simulink model "bh_2dof_STARTING_POINT_MODEL_SIMULINK"  (R2017a)
settings: Solver=ode45  StartTime=0.0  StopTime=20  RelTol=1e-5  EnableMultiTasking=on
settings Model: Creator=bhorton  LastModifiedBy=bhorton
settings OptimizationCC: LifeSpan=inf
settings DebuggingCC: SFUnexpectedBacktrackingDiag=warning  SFNoUnconditionalDefaultTransitionDiag=warning  SFExecutionAtInitializationDiag=none
settings GRTTargetCC: TargetLangStandard=C89/C90 (ANSI)  GeneratePreprocessorConditionals=Disable all
settings ConfigComp: CovMetricSettings=dw  CovHtmlReporting=on  CovSaveCumulativeToWorkspaceVar=on  CovSaveSingleToWorkspaceVar=on  CovExternalEMLEnable=off

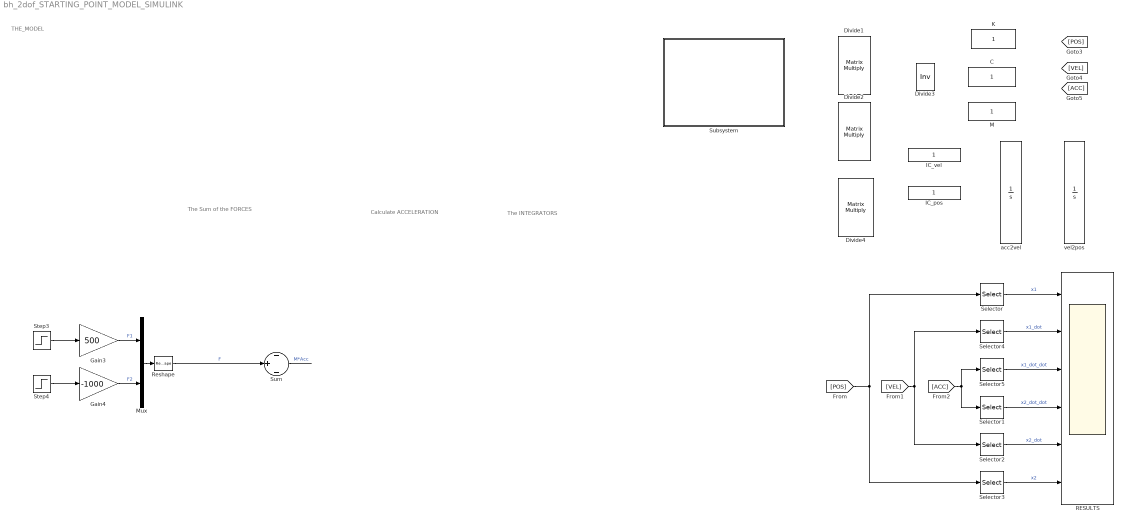
== system bh_2dof_STARTING_POINT_MODEL_SIMULINK ==
  note: The Sum of the FORCES
  note: Calculate ACCELERATION
  note: The INTEGRATORS
  note: THE_MODEL
  C : Constant
  Divide1 : Product  Multiplication=Matrix(*)
  Divide2 : Product  Multiplication=Matrix(*)
  Divide3 : Product  Inputs=/  Multiplication=Matrix(*)
  Divide4 : Product  Multiplication=Matrix(*)
  Gain3 : Gain  Gain=500
  Gain4 : Gain  Gain=-1000
  IC_pos : Constant
  IC_vel : Constant
  K : Constant
  M : Constant
  Mux : Mux  Inputs=2
  RESULTS : Scope  NumInputPorts=6
  Reshape : Reshape  OutputDimensionality=Column vector (2-D)
  Selector : Selector  InputPortWidth=2  IndexOptions=Index vector (dialog)  Indices=[1 ]  OutputSizes=1
  Selector1 : Selector  InputPortWidth=2  IndexOptions=Index vector (dialog)  Indices=[2]  OutputSizes=1
  Selector2 : Selector  InputPortWidth=2  IndexOptions=Index vector (dialog)  Indices=[2]  OutputSizes=1
  Selector3 : Selector  InputPortWidth=2  IndexOptions=Index vector (dialog)  Indices=[2]  OutputSizes=1
  Selector4 : Selector  InputPortWidth=2  IndexOptions=Index vector (dialog)  Indices=[1 ]  OutputSizes=1
  Selector5 : Selector  InputPortWidth=2  IndexOptions=Index vector (dialog)  Indices=[1 ]  OutputSizes=1
  Step3 : Step  Time=5  SampleTime=0
      settings: AttributesFormatString=Step @ T=%<Time>
  Step4 : Step  Time=10  SampleTime=0
      settings: AttributesFormatString=Step @ T=%<Time>
  Subsystem : Subsystem
      mask init:
      | str1 = 'Double click me';
      | str2 = 'to load MODEL';
      | str3 = 'parameters into';
      | str4 = 'Workspace';
      settings: OpenFcn=|
      | clc;
      | bh_script_2dof_params;
      | whos
      | fprintf('\n %s', repmat('#',1,70));
      | fprintf('\n DONE ! \n')
      mask Display: fprintf('%s\n%s\n%s\n%s',str1,str2,str3,str4)
  Sum : Sum  Inputs=-|+|-
  acc2vel : Integrator  InitialConditionSource=external
  vel2pos : Integrator  InitialConditionSource=external
  wires:
  Selector4/1 -> RESULTS/2  "x1_dot"
  [ACC] -> Selector5/1, Selector1/1
  Selector5/1 -> RESULTS/3  "x1_dot_dot"
  Selector/1 -> RESULTS/1  "x1"
  Mux/1 -> Reshape/1
  Reshape/1 -> Sum/2  "F"
  Selector3/1 -> RESULTS/6  "x2"
  [VEL] -> Selector4/1, Selector2/1
  Selector1/1 -> RESULTS/4  "x2_dot_dot"
  [POS] -> Selector/1, Selector3/1
  Selector2/1 -> RESULTS/5  "x2_dot"
  Step3/1 -> Gain3/1
  Step4/1 -> Gain4/1
  Gain3/1 -> Mux/1  "F1"
  Gain4/1 -> Mux/2  "F2"
  Sum/1 -> ?  "M*Acc"

== system bh_2dof_STARTING_POINT_MODEL_SIMULINK/Subsystem ==
